simulink model "CWE150_harness"  (R2018a)
settings: Solver=FixedStepAuto  StartTime=0  StopTime=20  FixedStep=0.01  RelTol=1e-3
undefined symbols (not defined in the file): sigbuilder_block
settings Model: SldvGeneratedHarnessModel=TestUnitModel=CWE150|  Creator=aarrieta  LastModifiedBy=umarkiegi
settings DataIOCC: ExternalInput=externalinputdata  SaveFormat=StructureWithTime
settings OptimizationCC: LifeSpan=inf
settings DebuggingCC: UnderspecifiedInitializationDetection=Classic  MergeDetectMultiDrivingBlocksExec=none  SolverPrmCheckMsg=warning  InheritedTsInSrcMsg=none  StateNameClashWarn=warning  SFUnexpectedBacktrackingDiag=warning  SFNoUnconditionalDefaultTransitionDiag=warning  SFExecutionAtInitializationDiag=none
settings HardwareCC: ProdBitPerPointer=32  ProdBitPerSizeT=32  ProdBitPerPtrDiffT=32  ProdLargestAtomicFloat=None  ProdIntDivRoundTo=Undefined  ProdEndianess=Unspecified  ProdWordSize=32  ProdHWDeviceType=32-bit Generic
settings ModelReferenceCC: PropagateSignalLabelsOutOfModel=off
settings CodeAppCC: StateflowObjectComments=on
settings GRTTargetCC: TargetLangStandard=C89/C90 (ANSI)  GeneratePreprocessorConditionals=Disable all
settings ConfigComp: CovEnable=on  CovScope=ReferencedModels  RecordCoverage=on  CovMetricSettings=dcmobe  CovHTMLOptions=-aTS=1 -bRG=1 -bTC=0 -hTR=0 -nFC=0 -scm=1 -bcm=1  CovHtmlReporting=on  CovSaveCumulativeToWorkspaceVar=on  CovSaveSingleToWorkspaceVar=on  DVMaxTestCaseSteps=20  DVTestSuiteOptimization=CombinedObjectives (Nonlinear Extended)  DVDetectFloatOverflow=off

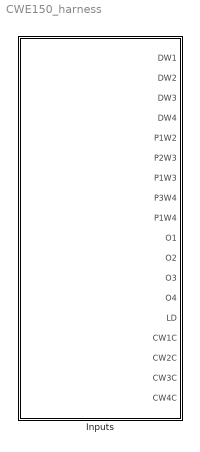
== system CWE150_harness ==
  Inputs : Subsystem  Tag=STV Subsys  LoadFcn=sigbuilder_block('load');  StartFcn=sigbuilder_block('start');  StopFcn=sigbuilder_block('stop');  ClipboardFcn=sigbuilder_block('clipboard');  mask(Sigbuilder block){tuvar=[0:10]}
      mask init:
      | if ~strcmp(get_param(bdroot(gcb),'SimulationStatus'),'stopped'),tuvar = sigbuilder_block('maskInit'); end
      settings: CopyFcn=sigbuilder_block('copy');  DeleteFcn=sigbuilder_block('delete');  ModelCloseFcn=sigbuilder_block('modelClose');  PreSaveFcn=sigbuilder_block('preSave');  PauseFcn=sigbuilder_block('pause');  ContinueFcn=sigbuilder_block('continue');  NameChangeFcn=sigbuilder_block('namechange');  OpenFcn=sigbuilder_block('open',[50 50 520 400 ]);  CloseFcn=sigbuilder_block('close');
      mask Display: plot(0, 0, 100, 100,[2, 2, 32, 32, 2], [68, 8, 8, 68, 68],[32, 2], [38, 38], [32, 19, 2],[53, 60, 44], [32, 17, 17, 2],[16, 16, 31, 31]);txt = getActiveGroup(gcbh);text(2, 100, txt,'verticalAlignment', 'top');

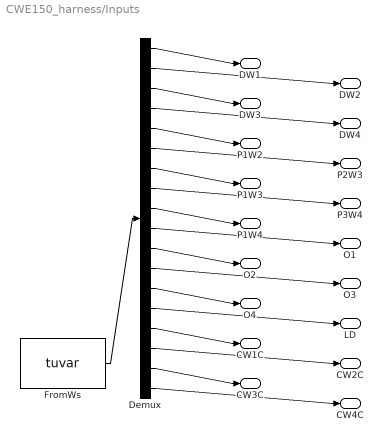
== system CWE150_harness/Inputs ==
  Demux : Demux  Tag=STV Demux  Outputs=18
  FromWs : FromWorkspace  Tag=STV FromWs  VariableName=tuvar  SampleTime=0
  DW1 : Outport  Tag=STV Outport
  DW2 : Outport  Tag=STV Outport  Port=2
  DW3 : Outport  Tag=STV Outport  Port=3
  DW4 : Outport  Tag=STV Outport  Port=4
  P1W2 : Outport  Tag=STV Outport  Port=5
  P2W3 : Outport  Tag=STV Outport  Port=6
  P1W3 : Outport  Tag=STV Outport  Port=7
  P3W4 : Outport  Tag=STV Outport  Port=8
  P1W4 : Outport  Tag=STV Outport  Port=9
  O1 : Outport  Tag=STV Outport  Port=10
  O2 : Outport  Tag=STV Outport  Port=11
  O3 : Outport  Tag=STV Outport  Port=12
  O4 : Outport  Tag=STV Outport  Port=13
  LD : Outport  Tag=STV Outport  Port=14
  CW1C : Outport  Tag=STV Outport  Port=15
  CW2C : Outport  Tag=STV Outport  Port=16
  CW3C : Outport  Tag=STV Outport  Port=17
  CW4C : Outport  Tag=STV Outport  Port=18
  wires:
  FromWs/1 -> Demux/1
  Demux/1 -> DW1/1
  Demux/2 -> DW2/1
  Demux/3 -> DW3/1
  Demux/4 -> DW4/1
  Demux/5 -> P1W2/1
  Demux/6 -> P2W3/1
  Demux/7 -> P1W3/1
  Demux/8 -> P3W4/1
  Demux/9 -> P1W4/1
  Demux/10 -> O1/1
  Demux/11 -> O2/1
  Demux/12 -> O3/1
  Demux/13 -> O4/1
  Demux/14 -> LD/1
  Demux/15 -> CW1C/1
  Demux/16 -> CW2C/1
  Demux/17 -> CW3C/1
  Demux/18 -> CW4C/1
